simulink model "pmsm_foc_sensorless_nucleo_G4"  (R2024a)
settings: Solver=FixedStepDiscrete  StartTime=0.0  StopTime=inf  RelTol=1e-3  EnableMultiTasking=on
InitFcn:
  | stm32_pmsm_foc_data;
model workspace (MAT data in the model file):
  encoderResolution = 2000
  hallOffset = '0.5'
  indexOffset = 850
  polePairs = '4'
undefined symbols (not defined in the file): PWM_frequency
libraries: mcbcontrolslib x7, stm32f4xxblockslib x3, simulink x2, slpidlib x2, stm32g4xxblockslib x2, stm32blockslib x2, mcbsensorlessestimatorlib x1
settings Model: SimulationMode=external  CodeVerificationMode=processor-in-the-loop (pil)  Creator=The MathWorks, Inc.  LastModifiedBy=wsl
settings SolverCC: AlgebraicLoopSolver=TrustRegion  AutoInsertRateTranBlk=on
settings DataIOCC: LimitDataPoints=on  SaveFormat=Array  SaveOutput=off  SaveTime=off  ReturnWorkspaceOutputs=off
settings OptimizationCC: DefaultUnderspecifiedDataType=single  OptimizeBlockIOStorage=off  BufferReuse=off  ReuseModelBlockBuffer=off  GlobalBufferReuse=off  ExpressionFolding=off  ExpressionDepthLimit=2147483647  LocalBlockOutputs=off  ZeroExternalMemoryAtStartup=off  InitFltsAndDblsToZero=on  EfficientFloat2IntCast=on  LifeSpan=Inf  MaxStackSize=64  OptimizeDataStoreBuffers=off  BusAssignmentInplaceUpdate=off  EfficientTunableParamExpr=on
settings DebuggingCC: ReadBeforeWriteMsg=DisableAll  WriteAfterWriteMsg=DisableAll  WriteAfterReadMsg=DisableAll  CheckSSInitialOutputMsg=off  SolverPrmCheckMsg=warning  InheritedTsInSrcMsg=none  MultiTaskDSMMsg=none  MultiTaskCondExecSysMsg=none  TasksWithSamePriorityMsg=none  SigSpecEnsureSampleTimeMsg=none  IntegerOverflowMsg=none  ParameterPrecisionLossMsg=none  FcnCallInpInsideContextMsg=warning  UnconnectedInputMsg=warning  UnconnectedOutputMsg=warning  UnconnectedLineMsg=warning  AllowSymbolicDim=off  StateNameClashWarn=warning  SubsystemReferenceDiagnosticForUnitTest=warning  SFUnexpectedBacktrackingDiag=warning  SFNoUnconditionalDefaultTransitionDiag=warning  SFExecutionAtInitializationDiag=none  IntegerSaturationMsg=none  ArithmeticOperatorsInVariantConditions=warning
settings HardwareCC: ProdBitPerPointer=32  ProdBitPerSizeT=32  ProdBitPerPtrDiffT=32  ProdLargestAtomicInteger=Long  ProdLargestAtomicFloat=Double  ProdWordSize=32  ProdLongLongMode=on  ProdHWDeviceType=ARM Compatible->ARM Cortex-M  TargetBitPerChar=16  TargetBitPerInt=16  TargetBitPerPointer=16  TargetLargestAtomicInteger=Integer  TargetIntDivRoundTo=Zero  TargetEndianess=LittleEndian  TargetWordSize=16  TargetHWDeviceType=TI C2000
settings ModelReferenceCC: EnableRefExpFcnMdlSchedulingChecks=on  PropagateSignalLabelsOutOfModel=off
settings SFSimCC: SimUseLocalCustomCode=off  SimParseCustomCode=off  MATLABDynamicMemAlloc=off  CustomCodeUndefinedFunction=UseInterfaceOnly
settings RTWCC: Description=Embedded Coder  SystemTargetFile=ert.tlc  HardwareBoard=STM32G4xx Based  TemplateMakefile=ert_default_tmf  RTWUseLocalCustomCode=off  Toolchain=GNU Tools for ARM Embedded Processors  BuildConfiguration=Faster Runs  IncludeHyperlinkInReport=on  GPUComputeCapability=3.5  DLArmComputeVersion=19.05
settings CodeAppCC: IgnoreCustomStorageClasses=off  CustomSymbolStrType=$N$R$M  StateflowObjectComments=on  InternalIdentifier=Classic
settings ERTTargetCC: TargetLangStandard=C99 (ISO)  CodeReplacementLibrary=ARM Cortex-M  MultiwordLength=2048  SupportVariableSizeSignals=on  ExtModeTransport=3  ExtModeStaticAlloc=on  ExtModeStaticAllocSize=2048  ExtModeMexFile=ext_xcp  ExtModeIntrfLevel=Level2 - Open  ConvertIfToSwitch=off  SuppressUnreachableDefaultCases=off
settings ConfigComp: CovMetricSettings=dw  CovSaveCumulativeToWorkspaceVar=on  CovSaveSingleToWorkspaceVar=on  CovExternalEMLEnable=off  CovSFcnEnable=off

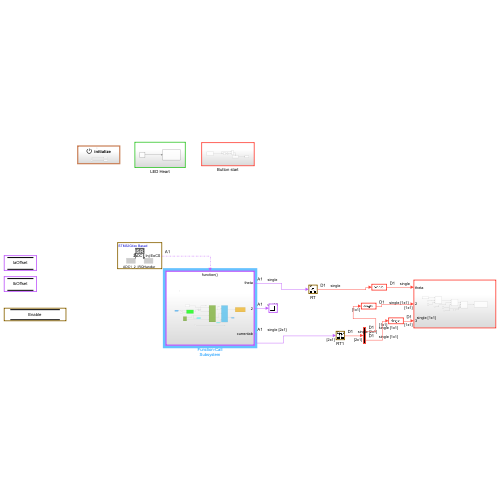
[thumbnail: Simulink's stored preview of the top-level diagram]
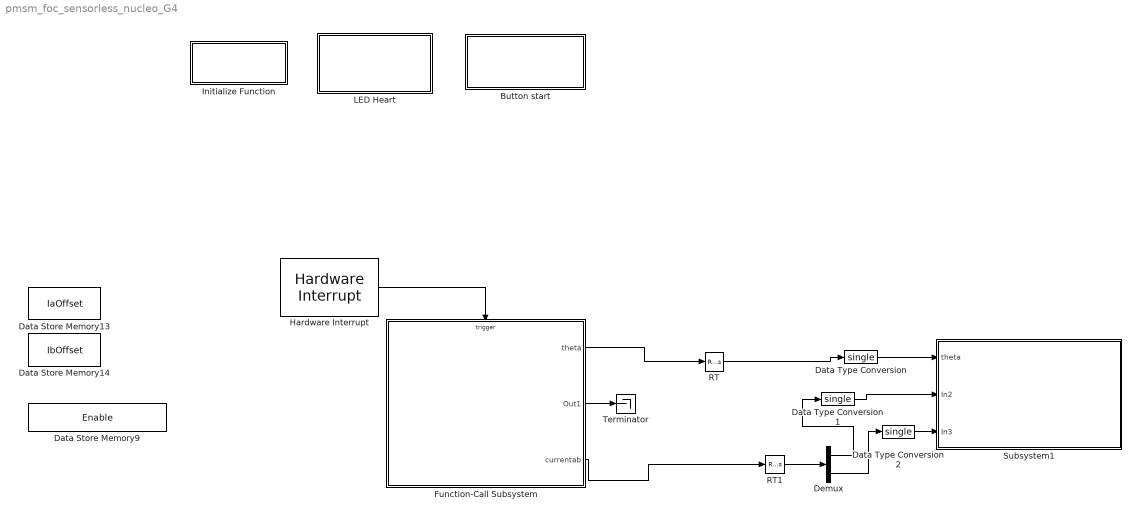
== system pmsm_foc_sensorless_nucleo_G4 ==
  Button start : Subsystem
  Data Store Memory13 : DataStoreMemory  DataStoreName=IaOffset  WriteAfterWriteMsg=warning  ShowAdditionalParam=off  OutDataTypeStr=int16
  Data Store Memory14 : DataStoreMemory  DataStoreName=IbOffset  WriteAfterWriteMsg=warning  ShowAdditionalParam=off  OutDataTypeStr=int16
  Data Store Memory9 : DataStoreMemory  DataStoreName=Enable  WriteAfterWriteMsg=warning  ShowAdditionalParam=off
  Data Type Conversion : DataTypeConversion  OutDataTypeStr=single  SaturateOnIntegerOverflow=off  RndMeth=Floor
  Data Type Conversion1 : DataTypeConversion  OutDataTypeStr=single  SaturateOnIntegerOverflow=off  RndMeth=Floor
  Data Type Conversion2 : DataTypeConversion  OutDataTypeStr=single  SaturateOnIntegerOverflow=off  RndMeth=Floor
  Demux : Demux  Outputs=2
  Function-Call Subsystem : Subsystem  TreatAsAtomicUnit=on
  Hardware Interrupt : stm32g4xxblockslib/Hardware Interrupt  ISRGroup=Analog to digital converter (ADC)  ISRName=ADC1_2_IRQHandler  ISRNumber=33  EventsList={ 'off', 'ADC1 OVR', '1'; 'off', 'ADC1 Reg EoCS', '2'; 'on', 'ADC1 Inj EoCS', '3'; 'off', 'ADC1 Inj JQOVF', '4'; 'off', 'ADC1 Watchdog1', '5'; 'off', 'ADC1 Watchdog2', '6'; 'off', 'ADC1 Watchdog3', '7'; 'off', 'ADC2 OVR', '8'; 'off', 'ADC2 Reg EoCS', '9'; 'off', 'ADC2 Inj EoCS', '10'; 'off', 'ADC2 Inj JQOVF', '11'; 'off', 'ADC2 Watchdog', '12'; 'off', 'ADC2 Watchdog2', '13'; 'off', 'ADC2 Watchdog3', '14'; 'off', 'Custom event', '15' }  SelectedEvents={'ADC1 Inj EoCS'}  TaskPriority=33  DisablePreemption=on  ClearInterruptFlagsAtEndOfEvent=off  InterruptDefinitionFile=$(TARGET_ROOT)/registry/interrupts/STM32F4xxBased_interrupts.xml  HardwareBoard=STM32G4xx Based  EnableSimPort=off
  Initialize Function : Subsystem  TreatAsAtomicUnit=on
  LED Heart : Subsystem
  RT : RateTransition  Deterministic=off  OutPortSampleTime=1e-3
  RT1 : RateTransition  Deterministic=off  OutPortSampleTime=1e-3
  Subsystem1 : Subsystem
  Terminator : Terminator
  wires:
  Hardware Interrupt/1 -> Function-Call Subsystem/Trigger
  RT/1 -> Data Type Conversion/1
  Demux/2 -> Data Type Conversion2/1
  Demux/1 -> Data Type Conversion1/1
  Function-Call Subsystem/3(currentab) -> RT1/1
  Data Type Conversion/1 -> Subsystem1/1(theta)
  Data Type Conversion1/1 -> Subsystem1/2(In2)
  Data Type Conversion2/1 -> Subsystem1/3(In3)
  Function-Call Subsystem/1(theta) -> RT/1
  RT1/1 -> Demux/1
  Function-Call Subsystem/2(Out1) -> Terminator/1

== system pmsm_foc_sensorless_nucleo_G4/Button start ==
  AND : Logic  AllPortsSameDT=off  OutDataTypeStr=boolean
  Data Store Write : DataStoreWrite  DataStoreName=Enable  IndexOptions=Index vector (dialog)  Indices=1  OutputSizes=1
  Digital Port Read : stm32f4xxblockslib/Digital Port Read  PortName=GPIOC  PinNumber=[13]  ReadOperation=on  IOAsArray=on  SampleTime=-1  EnableSimPort=off
      settings: LibrarySourceBlock=stm32g4xxblockslib/Digital Port Read
  Enabled Subsystem : Subsystem  TreatAsAtomicUnit=on
  NOT2 : Logic  Operator=NOT  IconShape=distinctive  AllPortsSameDT=off  OutDataTypeStr=boolean
  Unit Delay : UnitDelay  InitialCondition=false  SampleTime=-1  HasFrameUpgradeWarning=on
  wires:
  Enabled Subsystem/1(Out1) -> Data Store Write/1
  Digital Port Read/1 -> Unit Delay/1, AND/1
  NOT2/1 -> AND/2
  AND/1 -> Enabled Subsystem/Enable
  Unit Delay/1 -> NOT2/1

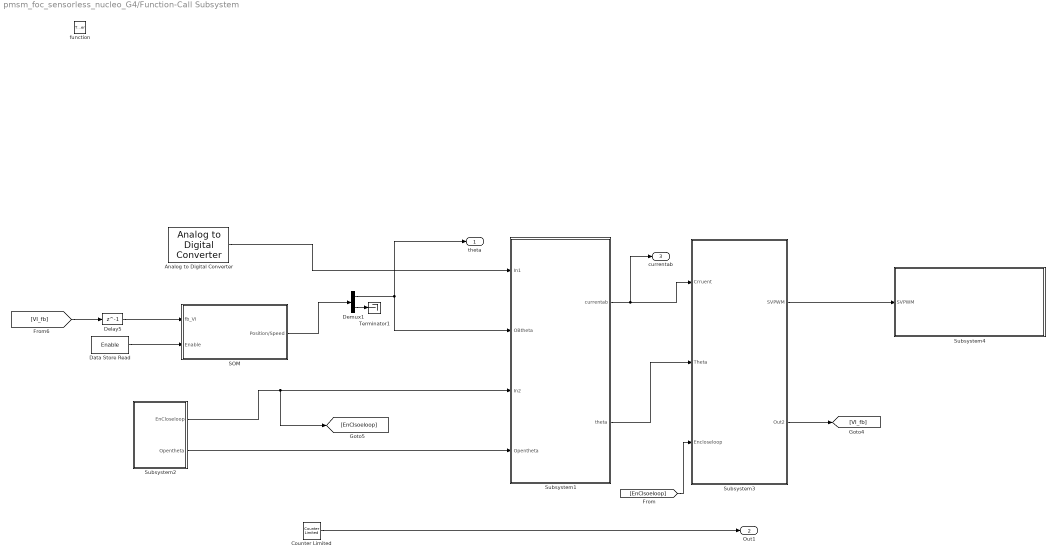
== system pmsm_foc_sensorless_nucleo_G4/Function-Call Subsystem ==
  function : TriggerPort  TriggerType=function-call  VariantControl=(inherit)
  Analog to Digital Converter : stm32f4xxblockslib/Analog to Digital Converter  ADCModule=ADC1  ConversionGroup=Injected  TriggerMode=Read results only  NumberOfConversions=2  EnableBufferConv=off  BufferLength=1  OutputStatus=off  SampleTime=-1  EnableSimPort=off
  Counter Limited : simulink/Sources/Counter Limited  uplimit=20000  tsamp=-1
  Data Store Read : DataStoreRead  DataStoreName=Enable  IndexOptions=Index vector (dialog)  Indices=1  OutputSizes=1
  Delay5 : Delay  DelayLength=1
  Demux1 : Demux  Outputs=2
  SOM : Subsystem
  Subsystem1 : Subsystem
  Subsystem2 : Subsystem
  Subsystem3 : Subsystem
  Subsystem4 : Subsystem
  Terminator1 : Terminator
  theta : Outport
  Out1 : Outport  Port=2
  currentab : Outport  Port=3
  wires:
  Subsystem1/1(currentab) -> currentab/1, Subsystem3/1(Crruent)
  Subsystem2/1(EnCloseloop) -> [EnClsoeloop], Subsystem1/3(In2)
  Subsystem2/2(Opentheta) -> Subsystem1/4(Opentheta)
  Demux1/2 -> Terminator1/1
  SOM/1(Position/Speed) -> Demux1/1
  Delay5/1 -> SOM/1(fb_VI)
  [VI_fb] -> Delay5/1
  Demux1/1 -> Subsystem1/2(OBtheta), theta/1
  Analog to Digital Converter/1 -> Subsystem1/1(In1)
  Subsystem1/2(theta) -> Subsystem3/2(Theta)
  Subsystem3/2(Out2) -> [VI_fb]
  Subsystem3/1(SVPWM) -> Subsystem4/1(SVPWM)
  Counter Limited/1 -> Out1/1
  [EnClsoeloop] -> Subsystem3/3(Encloseloop)
  Data Store Read/1 -> SOM/2(Enable)

== system pmsm_foc_sensorless_nucleo_G4/Initialize Function ==
  Data Store Write : DataStoreWrite  DataStoreName=IaOffset  IndexOptions=Index vector (dialog)  Indices=1  OutputSizes=1
  Data Store Write1 : DataStoreWrite  DataStoreName=IbOffset  IndexOptions=Index vector (dialog)  Indices=1  OutputSizes=1
  Event Listener : EventListener  DisableCoverage=on  EventName=reset
  Testing get offset : Constant  Value=2075  OutDataTypeStr=int16
  Testing get offset1 : Constant  Value=2051  OutDataTypeStr=int16
  wires:
  Testing get offset1/1 -> Data Store Write/1
  Testing get offset/1 -> Data Store Write1/1

== system pmsm_foc_sensorless_nucleo_G4/LED Heart ==
  Digital Port Write : stm32f4xxblockslib/Digital Port Write  PortName=GPIOA  PinNumber=[5]  ReadOperation=off  IOAsArray=on  EnableSimPort=off
      settings: LibrarySourceBlock=stm32g4xxblockslib/Digital Port Write
  Pulse Generator : DiscretePulseGenerator  Period=10  PulseWidth=5  SampleTime=0.1
  wires:
  Pulse Generator/1 -> Digital Port Write/1  "LED"

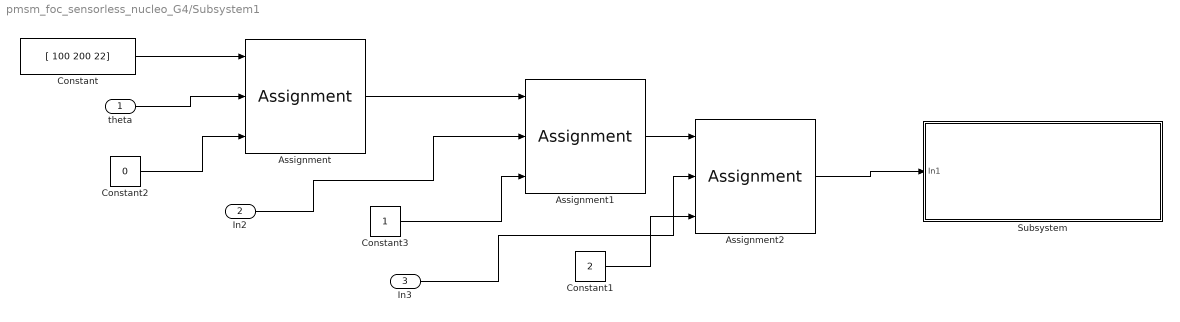
== system pmsm_foc_sensorless_nucleo_G4/Subsystem1 ==
  theta : Inport
  In2 : Inport  Port=2
  In3 : Inport  Port=3
  Assignment : Assignment  IndexMode=Zero-based  DiagnosticForDimensions=Warning  IndexOptions=Index vector (port)  Indices=2  OutputSizes=1
  Assignment1 : Assignment  IndexMode=Zero-based  DiagnosticForDimensions=Warning  IndexOptions=Index vector (port)  Indices=2  OutputSizes=1
  Assignment2 : Assignment  IndexMode=Zero-based  DiagnosticForDimensions=Warning  IndexOptions=Index vector (port)  Indices=2  OutputSizes=1
  Constant : Constant  Value=[ 100 200 22]  OutDataTypeStr=single
  Constant1 : Constant  Value=2  OutDataTypeStr=uint8
  Constant2 : Constant  Value=0  OutDataTypeStr=uint8
  Constant3 : Constant  OutDataTypeStr=uint8
  Subsystem : Subsystem
  wires:
  Constant/1 -> Assignment/1
  Assignment1/1 -> Assignment2/1
  theta/1 -> Assignment/2
  In3/1 -> Assignment2/2
  Assignment/1 -> Assignment1/1
  In2/1 -> Assignment1/2
  Assignment2/1 -> Subsystem/1(In1)
  Constant3/1 -> Assignment1/3
  Constant2/1 -> Assignment/3
  Constant1/1 -> Assignment2/3

== system pmsm_foc_sensorless_nucleo_G4/Button start/Enabled Subsystem ==
  Enable : EnablePort
  NOT : Logic  Operator=NOT  IconShape=distinctive  AllPortsSameDT=off  OutDataTypeStr=boolean
  Unit Delay : UnitDelay  InitialCondition=true  SampleTime=-1  HasFrameUpgradeWarning=on
  Out1 : Outport
  wires:
  Unit Delay/1 -> NOT/1, Out1/1
  NOT/1 -> Unit Delay/1

== system pmsm_foc_sensorless_nucleo_G4/Function-Call Subsystem/SOM ==
  fb_VI : Inport
  Enable : Inport  Port=2
  Demux1 : Demux
  Logical Operator : Logic  Operator=NOT  IconShape=distinctive  AllPortsSameDT=off  OutDataTypeStr=boolean
  Mux : Mux  Inputs=2
  Sliding Mode Observer : mcbsensorlessestimatorlib/Sliding Mode Observer  InputUnit=Per-unit  BlkSampleTime=1/PWM_frequency  StatorResistance=18.15  StatorInductance=0.0407  MaxApplicationSpeed=3000  PolePairs=2  MaxStatorVoltage=110/1.732  MaxStatorCurrent=1  DisturbanceObserverGain=0.9  CurrentObserverGain=0.0029627  CutoffFreq=300  PositionUnit=Per unit  PositionDataType=single  SpeedUnit=RPM  PerUnitSpeed=PU_System.N_base  SpeedDataType=single
  Position/Speed : Outport
  wires:
  Logical Operator/1 -> Sliding Mode Observer/5
  Mux/1 -> Position/Speed/1
  Demux1/3 -> Sliding Mode Observer/3  "Ialpha"
  fb_VI/1 -> Demux1/1
  Sliding Mode Observer/2 -> Mux/2
  Demux1/2 -> Sliding Mode Observer/2
  Sliding Mode Observer/1 -> Mux/1
  Enable/1 -> Logical Operator/1
  Demux1/1 -> Sliding Mode Observer/1
  Demux1/4 -> Sliding Mode Observer/4  "Ibeta"

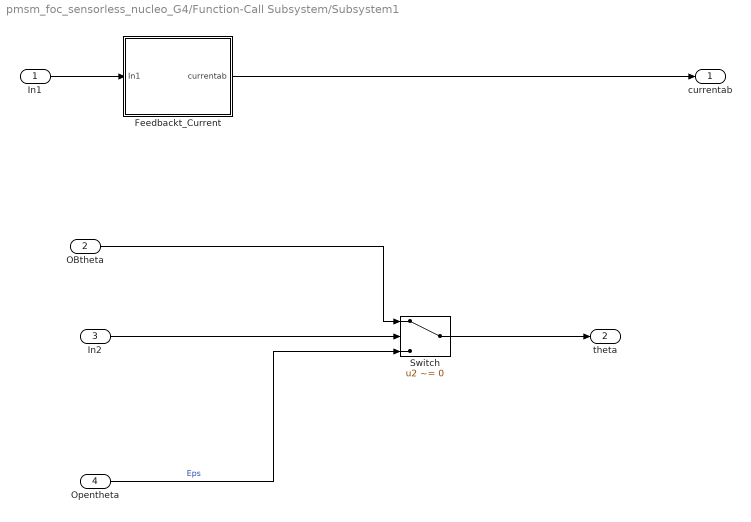
== system pmsm_foc_sensorless_nucleo_G4/Function-Call Subsystem/Subsystem1 ==
  In1 : Inport
  OBtheta : Inport  Port=2
  In2 : Inport  Port=3
  Opentheta : Inport  Port=4
  Feedbackt_Current : Subsystem
  Switch : Switch  Criteria=u2 ~= 0  Threshold=0.1  SaturateOnIntegerOverflow=off  InputSameDT=off
  currentab : Outport
  theta : Outport  Port=2
  wires:
  Opentheta/1 -> Switch/3  "Eps"
  In2/1 -> Switch/2
  Feedbackt_Current/1(currentab) -> currentab/1
  Switch/1 -> theta/1
  OBtheta/1 -> Switch/1
  In1/1 -> Feedbackt_Current/1(In1)

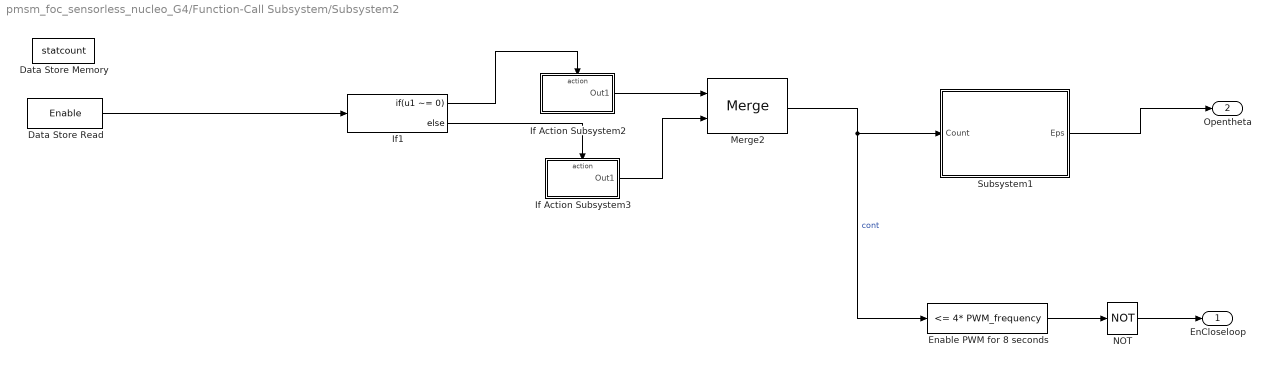
== system pmsm_foc_sensorless_nucleo_G4/Function-Call Subsystem/Subsystem2 ==
  Data Store Memory : DataStoreMemory  DataStoreName=statcount  WriteAfterWriteMsg=warning  ShowAdditionalParam=off
  Data Store Read : DataStoreRead  DataStoreName=Enable  IndexOptions=Index vector (dialog)  Indices=1  OutputSizes=1
  Enable PWM for 8 seconds : simulink/Logic and Bit Operations/Compare To Constant  relop=<=  const=4* PWM_frequency  OutDataTypeStr=boolean
  If Action Subsystem2 : Subsystem  TreatAsAtomicUnit=on
  If Action Subsystem3 : Subsystem  TreatAsAtomicUnit=on
  If1 : If  IfExpression=u1 ~= 0
  Merge2 : Merge
  NOT : Logic  Operator=NOT  IconShape=distinctive  AllPortsSameDT=off  OutDataTypeStr=boolean
  Subsystem1 : Subsystem
  EnCloseloop : Outport  OutputWhenDisabled=reset  InitialOutput=0  VectorParamsAs1DForOutWhenUnconnected=off
  Opentheta : Outport  Port=2
  wires:
  If1/2 -> If Action Subsystem3/Action
  If1/1 -> If Action Subsystem2/Action
  If Action Subsystem3/1(Out1) -> Merge2/2
  If Action Subsystem2/1(Out1) -> Merge2/1
  Merge2/1 -> Enable PWM for 8 seconds/1, Subsystem1/1(Count)  "cont"
  Data Store Read/1 -> If1/1
  NOT/1 -> EnCloseloop/1
  Subsystem1/1(Eps) -> Opentheta/1
  Enable PWM for 8 seconds/1 -> NOT/1

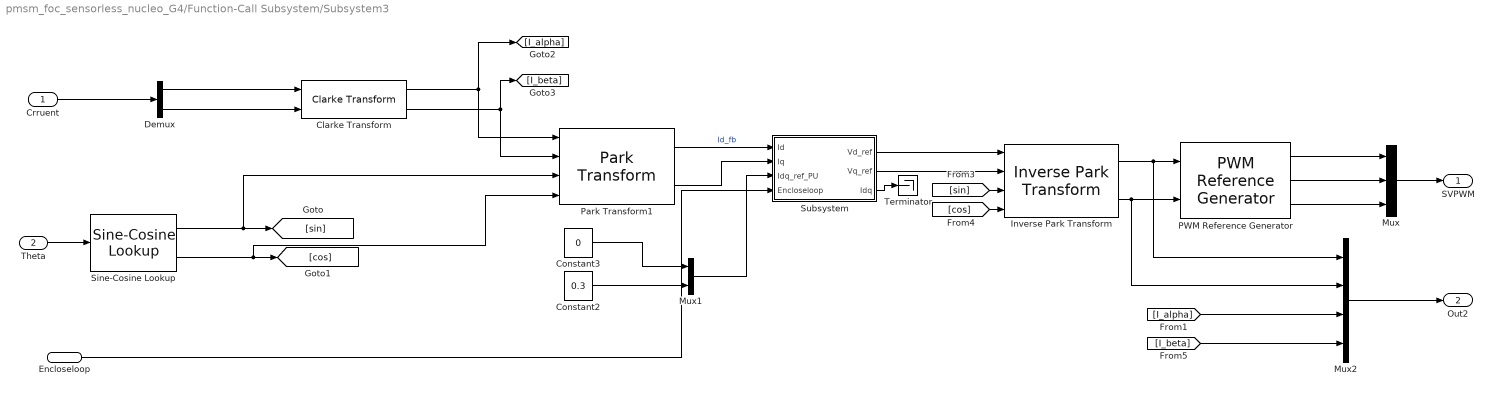
== system pmsm_foc_sensorless_nucleo_G4/Function-Call Subsystem/Subsystem3 ==
  Crruent : Inport
  Theta : Inport  Port=2
  Encloseloop : Inport  Port=3
  Clarke Transform : mcbcontrolslib/Clarke Transform  VariantControl=Variant2  PhaseInput=Two inputs  EnPowerInv=off
      settings: LibrarySourceBlock=mcbhdllib/Controls/Math Transforms/Clarke Transform
  Constant2 : Constant  Value=0.3  OutDataTypeStr=single
  Constant3 : Constant  Value=0  OutDataTypeStr=single
  Demux : Demux  Outputs=2
  Inverse Park Transform : mcbcontrolslib/Inverse Park Transform  PhaseInput=Two inputs  AxisAlignment=D-axis  ThetaInput=Sine and Cosine electrical position  AngleInput=Per-unit  N_points=1024
  Mux : Mux  Inputs=3
  Mux1 : Mux  Inputs=2
  Mux2 : Mux
  PWM Reference Generator : mcbcontrolslib/PWM Reference Generator  inSignal=Valphabeta  modType=SVM: space vector modulation
      settings: LibrarySourceBlock=mcblib/Controls/Math Transforms/PWM Reference Generator
  Park Transform1 : mcbcontrolslib/Park Transform  PhaseInput=Two inputs  AxisAlignment=D-axis  ThetaInput=Sine and Cosine electrical position  AngleInput=Per-unit  N_points=1024
      settings: LibrarySourceBlock=mcbhdllib/Controls/Math Transforms/Park Transform
  Sine-Cosine Lookup : mcbcontrolslib/Sine-Cosine Lookup  AngleInput=Per-unit  N_points=1024  DatatypeInput=Inherit from input  Datatype=single
  Subsystem : Subsystem
  Terminator : Terminator
  SVPWM : Outport
  Out2 : Outport  Port=2
  wires:
  Constant2/1 -> Mux1/2
  PWM Reference Generator/2 -> Mux/2
  Park Transform1/2 -> Subsystem/2(Iq)
  [cos] -> Inverse Park Transform/4
  Demux/2 -> Clarke Transform/2
  Sine-Cosine Lookup/1 -> Park Transform1/3, [sin]
  Subsystem/3(Idq) -> Terminator/1
  Demux/1 -> Clarke Transform/1
  Inverse Park Transform/1 -> Mux2/1, PWM Reference Generator/1
  Sine-Cosine Lookup/2 -> Park Transform1/4, [cos]
  Mux/1 -> SVPWM/1
  PWM Reference Generator/1 -> Mux/1
  Constant3/1 -> Mux1/1
  [sin] -> Inverse Park Transform/3
  Inverse Park Transform/2 -> Mux2/2, PWM Reference Generator/2
  [I_alpha] -> Mux2/3
  Clarke Transform/2 -> Park Transform1/2, [I_beta]
  Clarke Transform/1 -> Park Transform1/1, [I_alpha]
  Park Transform1/1 -> Subsystem/1(Id)  "Id_fb"
  [I_beta] -> Mux2/4
  Crruent/1 -> Demux/1
  PWM Reference Generator/3 -> Mux/3
  Mux1/1 -> Subsystem/3(Idq_ref_PU)
  Mux2/1 -> Out2/1
  Theta/1 -> Sine-Cosine Lookup/1
  Subsystem/1(Vd_ref) -> Inverse Park Transform/1
  Subsystem/2(Vq_ref) -> Inverse Park Transform/2
  Encloseloop/1 -> Subsystem/4(Encloseloop)

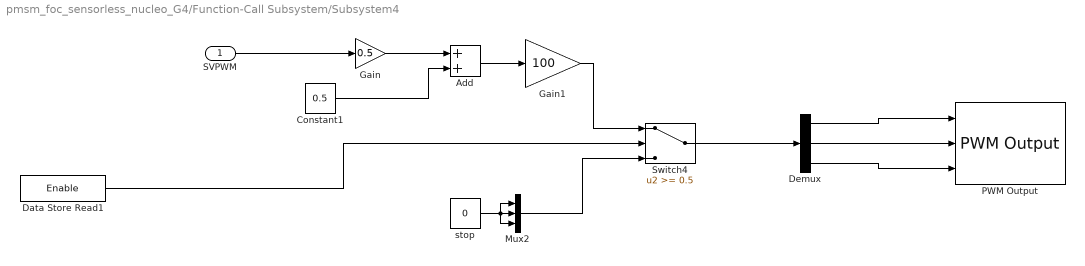
== system pmsm_foc_sensorless_nucleo_G4/Function-Call Subsystem/Subsystem4 ==
  SVPWM : Inport
  Add : Sum
  Constant1 : Constant  Value=0.5  OutDataTypeStr=single
  Data Store Read1 : DataStoreRead  DataStoreName=Enable  IndexOptions=Index vector (dialog)  Indices=1  OutputSizes=1
  Demux : Demux  Outputs=3
  Gain : Gain  Gain=0.5  OutDataTypeStr=single  RndMeth=Simplest
  Gain1 : Gain  Gain=100  OutDataTypeStr=single
  Mux2 : Mux  Inputs=3
  PWM Output : stm32g4xxblockslib/PWM Output  TimerModule=TIM1  DutycycleUnits=Percentage  EnableChannel1=on  EnableChannel2=on  EnableChannel3=on  EnableChannel4=off  EnableChannel5=off  EnableChannel6=off  EnableCounterInput=off  EnableMainOutputInput=off  EnableFrequencyInput=off  SetRCAfterCE=on  OutputDirection=off  OutputMainOutputEnableStatus=off  SampleTime=0.1  EnableSimPort=off  EnableUpdateEvent=off  EnableCaptureCompare1Event=off  EnableCaptureCompare2Event=off  EnableCaptureCompare3Event=off  EnableCaptureCompare4Event=off  EnableTriggerEvent=off  EnableBreakEvent=off  EnableBreakEvent2=off  ProcessorFamily=STM32G4  hoistedMaskSrc=ECSoC/ECSimCodegen/PWM Output
  Switch4 : Switch  Threshold=0.5  SaturateOnIntegerOverflow=off  InputSameDT=off
  stop : Constant  Value=0  OutDataTypeStr=uint16
  wires:
  Gain1/1 -> Switch4/1
  Gain/1 -> Add/1
  Add/1 -> Gain1/1
  Data Store Read1/1 -> Switch4/2
  stop/1 -> Mux2/2, Mux2/3, Mux2/1
  Constant1/1 -> Add/2
  SVPWM/1 -> Gain/1
  Switch4/1 -> Demux/1
  Mux2/1 -> Switch4/3
  Demux/2 -> PWM Output/2
  Demux/1 -> PWM Output/1
  Demux/3 -> PWM Output/3

== system pmsm_foc_sensorless_nucleo_G4/Subsystem1/Subsystem ==
  In1 : Inport
  Constant4 : Constant  Value=24  OutDataTypeStr=uint8
  Enabled Subsystem : Subsystem  TreatAsAtomicUnit=on
  NOT : Logic  Operator=NOT  IconShape=distinctive  AllPortsSameDT=off  OutDataTypeStr=boolean
  UART/USART Write : stm32blockslib/UART//USART Write  UARTModule=LPUART1  LengthOfDataToSend=on  BlockingMode=off  BlockingTimeout=0.1  OutputStatus=on
      settings: LibrarySourceBlock=stm32g4xxblockslib/UART//USART Write
  wires:
  Constant4/1 -> UART/USART Write/2
  In1/1 -> UART/USART Write/1
  UART/USART Write/1 -> NOT/1
  NOT/1 -> Enabled Subsystem/Enable

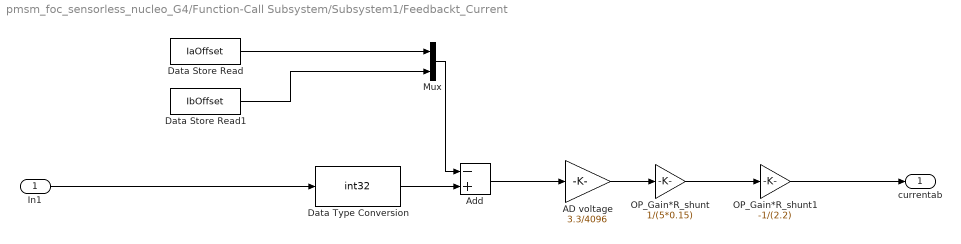
== system pmsm_foc_sensorless_nucleo_G4/Function-Call Subsystem/Subsystem1/Feedbackt_Current ==
  In1 : Inport
  AD voltage : Gain  Gain=3.3/4096  ParamDataTypeStr=single
  Add : Sum  Inputs=-+
  Data Store Read : DataStoreRead  DataStoreName=IaOffset  IndexOptions=Index vector (dialog)  Indices=1  OutputSizes=1
  Data Store Read1 : DataStoreRead  DataStoreName=IbOffset  IndexOptions=Index vector (dialog)  Indices=1  OutputSizes=1
  Data Type Conversion : DataTypeConversion  OutDataTypeStr=int32  ConvertRealWorld=Stored Integer (SI)  RndMeth=Simplest  SaturateOnIntegerOverflow=off
  Mux : Mux  Inputs=2
  OP_Gain*R_shunt : Gain  Gain=1/(5*0.15)  ParamDataTypeStr=single
  OP_Gain*R_shunt1 : Gain  Gain=-1/(2.2)  ParamDataTypeStr=single
  currentab : Outport
  wires:
  Add/1 -> AD voltage/1
  AD voltage/1 -> OP_Gain*R_shunt/1
  Mux/1 -> Add/1
  Data Type Conversion/1 -> Add/2
  Data Store Read/1 -> Mux/1
  Data Store Read1/1 -> Mux/2
  In1/1 -> Data Type Conversion/1
  OP_Gain*R_shunt1/1 -> currentab/1
  OP_Gain*R_shunt/1 -> OP_Gain*R_shunt1/1

== system pmsm_foc_sensorless_nucleo_G4/Function-Call Subsystem/Subsystem2/If Action Subsystem2 ==
  Action Port : ActionPort  ActionPortLabel=if(u1 ~= 0)
  Add1 : Sum  SaturateOnIntegerOverflow=on
  Constant : Constant  OutDataTypeStr=uint32
  Data Store Read : DataStoreRead  DataStoreName=statcount  IndexOptions=Index vector (dialog)  Indices=1  OutputSizes=1
  Data Store Write : DataStoreWrite  DataStoreName=statcount  IndexOptions=Index vector (dialog)  Indices=1  OutputSizes=1
  Out1 : Outport
  wires:
  Add1/1 -> Data Store Write/1, Out1/1
  Data Store Read/1 -> Add1/2
  Constant/1 -> Add1/1

== system pmsm_foc_sensorless_nucleo_G4/Function-Call Subsystem/Subsystem2/If Action Subsystem3 ==
  Action Port : ActionPort  ActionPortLabel=else
  Constant15 : Constant  Value=0  OutDataTypeStr=uint32
  Data Store Write : DataStoreWrite  DataStoreName=statcount  IndexOptions=Index vector (dialog)  Indices=1  OutputSizes=1
  Out1 : Outport
  wires:
  Constant15/1 -> Out1/1, Data Store Write/1

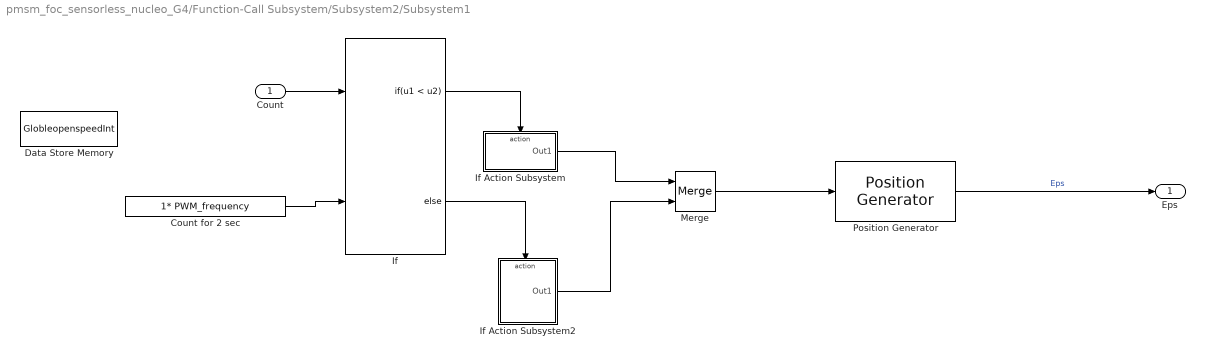
== system pmsm_foc_sensorless_nucleo_G4/Function-Call Subsystem/Subsystem2/Subsystem1 ==
  Count : Inport
  Count for 2 sec : Constant  Value=1* PWM_frequency  OutDataTypeStr=uint32  SampleTime=-1
  Data Store Memory : DataStoreMemory  DataStoreName=GlobleopenspeedInt  WriteAfterWriteMsg=warning  ShowAdditionalParam=off
  If : If  NumInputs=2  IfExpression=u1 < u2
  If Action Subsystem : Subsystem  TreatAsAtomicUnit=on
  If Action Subsystem2 : Subsystem  TreatAsAtomicUnit=on
  Merge : Merge
  Position Generator : mcbcontrolslib/Position Generator  AngleOutput=Per-unit  ExternalReset=none  Offset=0
  Eps : Outport
  wires:
  If Action Subsystem/1(Out1) -> Merge/1
  If/1 -> If Action Subsystem/Action
  If Action Subsystem2/1(Out1) -> Merge/2
  Count/1 -> If/1
  If/2 -> If Action Subsystem2/Action
  Count for 2 sec/1 -> If/2
  Merge/1 -> Position Generator/1
  Position Generator/1 -> Eps/1  "Eps"

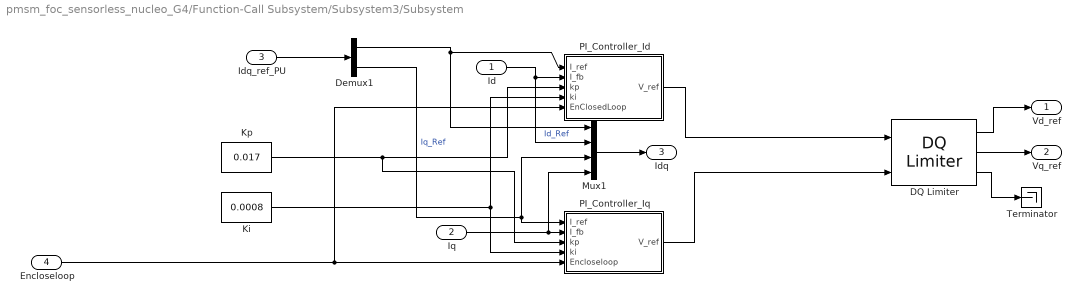
== system pmsm_foc_sensorless_nucleo_G4/Function-Call Subsystem/Subsystem3/Subsystem ==
  Id : Inport
  Iq : Inport  Port=2
  Idq_ref_PU : Inport  Port=3
  Encloseloop : Inport  Port=4
  DQ Limiter : mcbcontrolslib/DQ Limiter  satMethodInputType=Specify via dialog  satMethodSelected=D-Q equivalence  satLimitInputType=Specify via dialog  Vmax=0.95
  Demux1 : Demux  Outputs=2
  Ki : Constant  Value=0.0008  OutDataTypeStr=single  SampleTime=-1
  Kp : Constant  Value=0.017  OutDataTypeStr=single  SampleTime=-1
  Mux1 : Mux
  PI_Controller_Id : Subsystem
  PI_Controller_Iq : Subsystem
  Terminator : Terminator
  Vd_ref : Outport  VectorParamsAs1DForOutWhenUnconnected=off
  Vq_ref : Outport  Port=2  VectorParamsAs1DForOutWhenUnconnected=off
  Idq : Outport  Port=3  VectorParamsAs1DForOutWhenUnconnected=off
  wires:
  DQ Limiter/1 -> Vd_ref/1
  Demux1/2 -> Mux1/3, PI_Controller_Iq/1(I_ref)  "Iq_Ref"
  Id/1 -> Mux1/2, PI_Controller_Id/2(I_fb)
  Demux1/1 -> Mux1/1, PI_Controller_Id/1(I_ref)  "Id_Ref"
  Idq_ref_PU/1 -> Demux1/1
  Iq/1 -> Mux1/4, PI_Controller_Iq/2(I_fb)
  Mux1/1 -> Idq/1
  PI_Controller_Iq/1(V_ref) -> DQ Limiter/2
  DQ Limiter/2 -> Vq_ref/1
  PI_Controller_Id/1(V_ref) -> DQ Limiter/1
  DQ Limiter/3 -> Terminator/1
  Kp/1 -> PI_Controller_Id/3(kp), PI_Controller_Iq/3(kp)
  Ki/1 -> PI_Controller_Iq/4(ki), PI_Controller_Id/4(ki)
  Encloseloop/1 -> PI_Controller_Id/5(EnClosedLoop), PI_Controller_Iq/5(Encloseloop)

== system pmsm_foc_sensorless_nucleo_G4/Subsystem1/Subsystem/Enabled Subsystem ==
  Enable : EnablePort
  Constant1 : Constant  Value=[0 0 128 127 ]  OutDataTypeStr=uint8
  Constant2 : Constant  Value=4  OutDataTypeStr=uint8
  UART/USART Write : stm32blockslib/UART//USART Write  UARTModule=LPUART1  LengthOfDataToSend=on  BlockingMode=off  BlockingTimeout=0.1  OutputStatus=off
      settings: LibrarySourceBlock=stm32g4xxblockslib/UART//USART Write
  wires:
  Constant2/1 -> UART/USART Write/2
  Constant1/1 -> UART/USART Write/1

== system pmsm_foc_sensorless_nucleo_G4/Function-Call Subsystem/Subsystem2/Subsystem1/If Action Subsystem ==
  Action Port : ActionPort  ActionPortLabel=if(u1 < u2)
  Constant : Constant  Value=0  OutDataTypeStr=single
  Data Store Write : DataStoreWrite  DataStoreName=GlobleopenspeedInt  IndexOptions=Index vector (dialog)  Indices=1  OutputSizes=1
  Out1 : Outport
  wires:
  Constant/1 -> Out1/1, Data Store Write/1

== system pmsm_foc_sensorless_nucleo_G4/Function-Call Subsystem/Subsystem2/Subsystem1/If Action Subsystem2 ==
  Action Port : ActionPort  ActionPortLabel=else
  Add1 : Sum
  Constant2 : Constant  Value=1.5*(1/PWM_frequency)  VectorParams1D=off  OutDataTypeStr=single
  Data Store Read : DataStoreRead  DataStoreName=GlobleopenspeedInt  IndexOptions=Index vector (dialog)  Indices=1  OutputSizes=1
  Data Store Write : DataStoreWrite  DataStoreName=GlobleopenspeedInt  IndexOptions=Index vector (dialog)  Indices=1  OutputSizes=1
  Multiply1 : Gain  Gain=1/PWM_frequency  OutDataTypeStr=Inherit: Same as input
  Saturate to 'motor.calibSpeed' RPM : Saturate  UpperLimit=2 *120/60  LowerLimit=0
  Out1 : Outport
  wires:
  Constant2/1 -> Add1/1
  Saturate to 'motor.calibSpeed' RPM/1 -> Data Store Write/1, Multiply1/1
  Data Store Read/1 -> Add1/2
  Add1/1 -> Saturate to 'motor.calibSpeed' RPM/1
  Multiply1/1 -> Out1/1

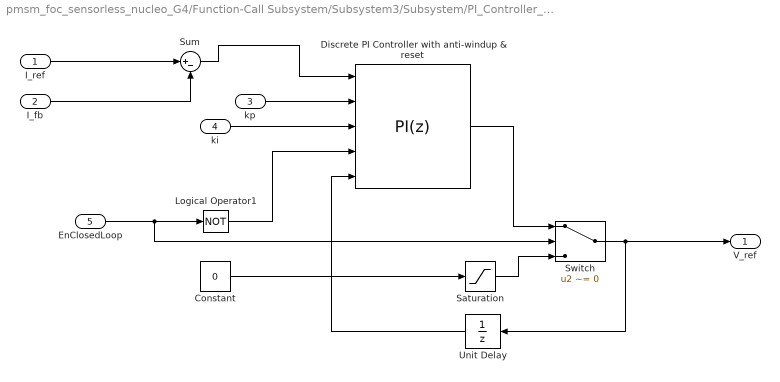
== system pmsm_foc_sensorless_nucleo_G4/Function-Call Subsystem/Subsystem3/Subsystem/PI_Controller_Id ==
  I_ref : Inport
  I_fb : Inport  Port=2
  kp : Inport  Port=3
  ki : Inport  Port=4
  EnClosedLoop : Inport  Port=5
  Constant : Constant  Value=0  OutDataTypeStr=single
  Discrete PI Controller with anti-windup & reset : slpidlib/PID Controller  Controller=PI  Form=Parallel  TimeDomain=Discrete-time  UseExternalTs=off  SampleTime=-1  IntegratorMethod=Forward Euler  FilterMethod=Forward Euler  ControllerParametersSource=external  P=1  I=1  UseKiTs=on  D=0  UseExternalDerivativeSource=off  N=100  UseFilter=on  TunerSelectOption=Transfer Function Based (PID Tuner App)  InitialConditionSource=external  InitialConditionForIntegrator=0  InitialConditionForFilter=0  DifferentiatorICPrevScaledInput=0  ExternalReset=level  TrackingMode=off  Kt=1  LimitOutput=on  SatLimitsSource=internal  UpperSaturationLimit=1  LowerSaturationLimit=-1  LinearizeAsGain=on  AntiWindupMode=clamping  Kb=1  LimitIntegrator=off  UpperIntegratorSaturationLimit=inf  LowerIntegratorSaturationLimit=-inf  RndMeth=Simplest  POutMin=[]  POutMax=[]  IOutMin=[]  IOutMax=[]  DOutMin=[]  DOutMax=[]  NOutMin=[]  NOutMax=[]  SumOutMin=[]  SumOutMax=[]  SaturationOutDataTypeStr=Inherit: Inherit via back propagation  SaturationOutMin=[]  SaturationOutMax=[]  PParamMin=[]  PParamMax=[]  IParamMin=[]  IParamMax=[]  DParamMin=[]  DParamMax=[]  NParamMin=[]  NParamMax=[]  KbParamMin=[]  KbParamMax=[]  KtParamMin=[]  KtParamMax=[]  KbOutMin=[]  KbOutMax=[]  KtOutMin=[]  KtOutMax=[]  IntegratorOutMin=[]  IntegratorOutMax=[]  FilterOutMin=[]  FilterOutMax=[]  SumI1OutMin=[]  SumI1OutMax=[]  SumI2OutMin=[]  SumI2OutMax=[]  SumI3OutMin=[]  SumI3OutMax=[]  SumI4OutMin=[]  SumI4OutMax=[]  SumDOutMin=[]  SumDOutMax=[]  DifferentiatorOutMin=[]  DifferentiatorOutMax=[]  FilterDiffOutCoefMin=[]  FilterDiffOutCoefMax=[]  ReciprocalOutMin=[]  ReciprocalOutMax=[]  SumDenOutMin=[]  SumDenOutMax=[]  SumNumOutMin=[]  SumNumOutMax=[]  DivideOutMin=[]  DivideOutMax=[]  UdiffTsProdOutMin=[]  UdiffTsProdOutMax=[]  NTsProdOutMin=[]  NTsProdOutMax=[]  UintegralTsProdOutMin=[]  UintegralTsProdOutMax=[]  UngainTsProdOutMin=[]  UngainTsProdOutMax=[]  ClampingZeroOutDataTypeStr=Inherit: Inherit via back propagation  ClampingZeroOutMin=[]  ClampingZeroOutMax=[]  FilterDenConstantOutDataTypeStr=Inherit: Inherit via back propagation  FilterDenConstantOutMin=[]  FilterDenConstantOutMax=[]  PCopyOutDataTypeStr=Inherit: Inherit via back propagation  PCopyOutMin=[]  PCopyOutMax=[]  NCopyOutDataTypeStr=Inherit: Inherit via back propagation  NCopyOutMin=[]  NCopyOutMax=[]  IntegratorContinuousStateAttributes=''  IntegratorStateMustResolveToSignalObject=off  IntegratorRTWStateStorageClass=Auto  FilterContinuousStateAttributes=''  FilterStateMustResolveToSignalObject=off  FilterRTWStateStorageClass=Auto  ParallelPVariant=ExternalParameters  IdealPVariant=Disabled  IVariant=ExternalParameters  DVariant=Disabled  IntegratorVariant=Discrete  SatVariant=Enabled  AWVariant=DiscClampingParallel  PCopyVariant=Disabled  TRVariant=Disabled  FdbkBlocksVariant=Forward  IdealPFdbkVariant=Disabled  SatFdbkVariant=Disabled  DerivativeFilterVariant=Disabled  NVariant=Disabled  NCopyVariant=Disabled_SignalSpec  FilterICVariant=Disabled  IntegratorICVariant=ExternalICs  ExternalResetVariant=ExternalReset  TRSumVariant=Passthrough  SumFdbkVariant=Disabled  SumVariant=Sum_PI  TsampFilterVariant=InternalTs  TsampNgainVariant=Passthrough  TsampIntegralVariant=Disabled_SignalSpec  ExternalSaturationOutDataTypeStr=Inherit: Same as second input  DerivativeSourceVariant=Disabled
      settings: LibrarySourceBlock=mcbcontrolslib/PI Controller
  Logical Operator1 : Logic  Operator=NOT  IconShape=distinctive  AllPortsSameDT=off  OutDataTypeStr=boolean
  Saturation : Saturate  RndMeth=Simplest
  Sum : Sum  Inputs=|+-  OutDataTypeStr=Inherit: Same as first input
  Switch : Switch  Criteria=u2 ~= 0  RndMeth=Simplest  SaturateOnIntegerOverflow=off  InputSameDT=off
  Unit Delay : UnitDelay  SampleTime=-1  HasFrameUpgradeWarning=on
  V_ref : Outport  VectorParamsAs1DForOutWhenUnconnected=off
  wires:
  I_ref/1 -> Sum/1
  I_fb/1 -> Sum/2
  Sum/1 -> Discrete PI Controller with anti-windup & reset/1
  Logical Operator1/1 -> Discrete PI Controller with anti-windup & reset/4
  kp/1 -> Discrete PI Controller with anti-windup & reset/2
  ki/1 -> Discrete PI Controller with anti-windup & reset/3
  Saturation/1 -> Switch/3
  EnClosedLoop/1 -> Logical Operator1/1, Switch/2
  Switch/1 -> V_ref/1, Unit Delay/1
  Discrete PI Controller with anti-windup & reset/1 -> Switch/1
  Constant/1 -> Saturation/1
  Unit Delay/1 -> Discrete PI Controller with anti-windup & reset/5

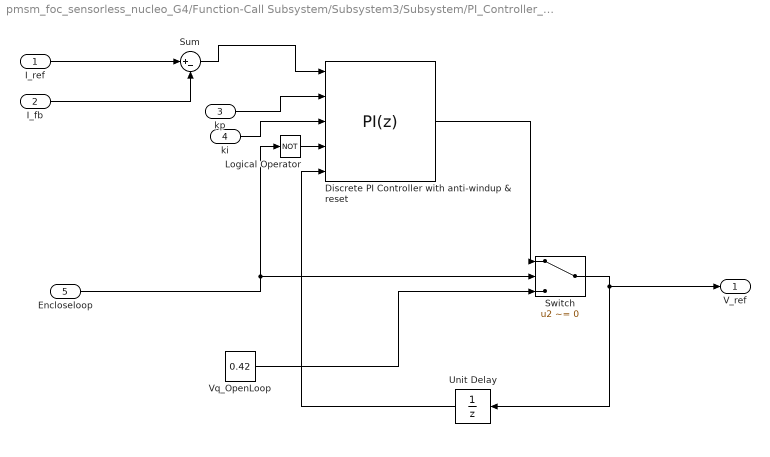
== system pmsm_foc_sensorless_nucleo_G4/Function-Call Subsystem/Subsystem3/Subsystem/PI_Controller_Iq ==
  I_ref : Inport
  I_fb : Inport  Port=2
  kp : Inport  Port=3
  ki : Inport  Port=4
  Encloseloop : Inport  Port=5
  Discrete PI Controller with anti-windup & reset : slpidlib/PID Controller  Controller=PI  Form=Parallel  TimeDomain=Discrete-time  UseExternalTs=off  SampleTime=-1  IntegratorMethod=Forward Euler  FilterMethod=Forward Euler  ControllerParametersSource=external  P=1  I=1  UseKiTs=on  D=0  UseExternalDerivativeSource=off  N=100  UseFilter=on  TunerSelectOption=Transfer Function Based (PID Tuner App)  InitialConditionSource=external  InitialConditionForIntegrator=0  InitialConditionForFilter=0  DifferentiatorICPrevScaledInput=0  ExternalReset=level  TrackingMode=off  Kt=1  LimitOutput=on  SatLimitsSource=internal  UpperSaturationLimit=1  LowerSaturationLimit=-1  LinearizeAsGain=on  AntiWindupMode=clamping  Kb=1  LimitIntegrator=off  UpperIntegratorSaturationLimit=inf  LowerIntegratorSaturationLimit=-inf  RndMeth=Simplest  POutMin=[]  POutMax=[]  IOutMin=[]  IOutMax=[]  DOutMin=[]  DOutMax=[]  NOutMin=[]  NOutMax=[]  SumOutMin=[]  SumOutMax=[]  SaturationOutDataTypeStr=Inherit: Inherit via back propagation  SaturationOutMin=[]  SaturationOutMax=[]  PParamMin=[]  PParamMax=[]  IParamMin=[]  IParamMax=[]  DParamMin=[]  DParamMax=[]  NParamMin=[]  NParamMax=[]  KbParamMin=[]  KbParamMax=[]  KtParamMin=[]  KtParamMax=[]  KbOutMin=[]  KbOutMax=[]  KtOutMin=[]  KtOutMax=[]  IntegratorOutMin=[]  IntegratorOutMax=[]  FilterOutMin=[]  FilterOutMax=[]  SumI1OutMin=[]  SumI1OutMax=[]  SumI2OutMin=[]  SumI2OutMax=[]  SumI3OutMin=[]  SumI3OutMax=[]  SumI4OutMin=[]  SumI4OutMax=[]  SumDOutMin=[]  SumDOutMax=[]  DifferentiatorOutMin=[]  DifferentiatorOutMax=[]  FilterDiffOutCoefMin=[]  FilterDiffOutCoefMax=[]  ReciprocalOutMin=[]  ReciprocalOutMax=[]  SumDenOutMin=[]  SumDenOutMax=[]  SumNumOutMin=[]  SumNumOutMax=[]  DivideOutMin=[]  DivideOutMax=[]  UdiffTsProdOutMin=[]  UdiffTsProdOutMax=[]  NTsProdOutMin=[]  NTsProdOutMax=[]  UintegralTsProdOutMin=[]  UintegralTsProdOutMax=[]  UngainTsProdOutMin=[]  UngainTsProdOutMax=[]  ClampingZeroOutDataTypeStr=Inherit: Inherit via back propagation  ClampingZeroOutMin=[]  ClampingZeroOutMax=[]  FilterDenConstantOutDataTypeStr=Inherit: Inherit via back propagation  FilterDenConstantOutMin=[]  FilterDenConstantOutMax=[]  PCopyOutDataTypeStr=Inherit: Inherit via back propagation  PCopyOutMin=[]  PCopyOutMax=[]  NCopyOutDataTypeStr=Inherit: Inherit via back propagation  NCopyOutMin=[]  NCopyOutMax=[]  IntegratorContinuousStateAttributes=''  IntegratorStateMustResolveToSignalObject=off  IntegratorRTWStateStorageClass=Auto  FilterContinuousStateAttributes=''  FilterStateMustResolveToSignalObject=off  FilterRTWStateStorageClass=Auto  ParallelPVariant=ExternalParameters  IdealPVariant=Disabled  IVariant=ExternalParameters  DVariant=Disabled  IntegratorVariant=Discrete  SatVariant=Enabled  AWVariant=DiscClampingParallel  PCopyVariant=Disabled  TRVariant=Disabled  FdbkBlocksVariant=Forward  IdealPFdbkVariant=Disabled  SatFdbkVariant=Disabled  DerivativeFilterVariant=Disabled  NVariant=Disabled  NCopyVariant=Disabled_SignalSpec  FilterICVariant=Disabled  IntegratorICVariant=ExternalICs  ExternalResetVariant=ExternalReset  TRSumVariant=Passthrough  SumFdbkVariant=Disabled  SumVariant=Sum_PI  TsampFilterVariant=InternalTs  TsampNgainVariant=Passthrough  TsampIntegralVariant=Disabled_SignalSpec  ExternalSaturationOutDataTypeStr=Inherit: Same as second input  DerivativeSourceVariant=Disabled
      settings: LibrarySourceBlock=mcbcontrolslib/PI Controller
  Logical Operator : Logic  Operator=NOT  IconShape=distinctive  AllPortsSameDT=off  OutDataTypeStr=boolean
  Sum : Sum  Inputs=|+-  OutDataTypeStr=Inherit: Same as first input
  Switch : Switch  Criteria=u2 ~= 0  RndMeth=Simplest  SaturateOnIntegerOverflow=off  InputSameDT=off
  Unit Delay : UnitDelay  SampleTime=-1  HasFrameUpgradeWarning=on
  Vq_OpenLoop : Constant  Value=0.42  OutDataTypeStr=single  SampleTime=-1
  V_ref : Outport  VectorParamsAs1DForOutWhenUnconnected=off
  wires:
  Encloseloop/1 -> Switch/2, Logical Operator/1
  I_fb/1 -> Sum/2
  I_ref/1 -> Sum/1
  Sum/1 -> Discrete PI Controller with anti-windup & reset/1
  Logical Operator/1 -> Discrete PI Controller with anti-windup & reset/4
  kp/1 -> Discrete PI Controller with anti-windup & reset/2
  ki/1 -> Discrete PI Controller with anti-windup & reset/3
  Discrete PI Controller with anti-windup & reset/1 -> Switch/1
  Vq_OpenLoop/1 -> Switch/3
  Switch/1 -> V_ref/1, Unit Delay/1
  Unit Delay/1 -> Discrete PI Controller with anti-windup & reset/5
